simulink library "RGP_regression"  (R2020a)
settings: Solver=VariableStepAuto  StartTime=0.0  StopTime=10.0  RelTol=1e-3
values from neighbouring files (symbols this model uses):
  basisCovMat = basisCovMat + tril(basisCovMat,-1)'    [RGP_regression_ts.m]
  basisVector = rgp.xBasis    [RGP_regression_ts.m]
  hyperParameters = [rgp.spatialCovAmp(:); rgp.spatialLengthScale(:)]    [RGP_regression_ts.m]
  meanFcnProperties = rgp.meanFnProps    [RGP_regression_ts.m]
  meanFcnVector = meanFunction(basisVector,0)    [RGP_regression_ts.m]
  noiseVariance = rgp.noiseVariance    [RGP_regression_ts.m]
libraries: dspsigops x2, dspmtrx3 x1
settings Model: Creator=Ayaz  LastModifiedBy=Ayaz

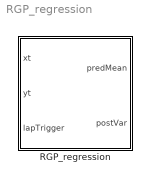
== system RGP_regression ==
  RGP_regression : Subsystem  mask{xBasis=basisVector, meanFcnProp=meanFcnProperties, meanFcnVec=meanFcnVector, hyperParams=hyperParameters, basisCovMat=basisCovMat, noiseVar=noiseVariance}
      mask prompts: xBasis "Basis vector"; meanFcnProp "Mean function properties"; meanFcnVec "Mean function vector"; hyperParams "Covariance hyperparameters"; basisCovMat "Basis vectors covariance matrix"; noiseVar "Noise variance"

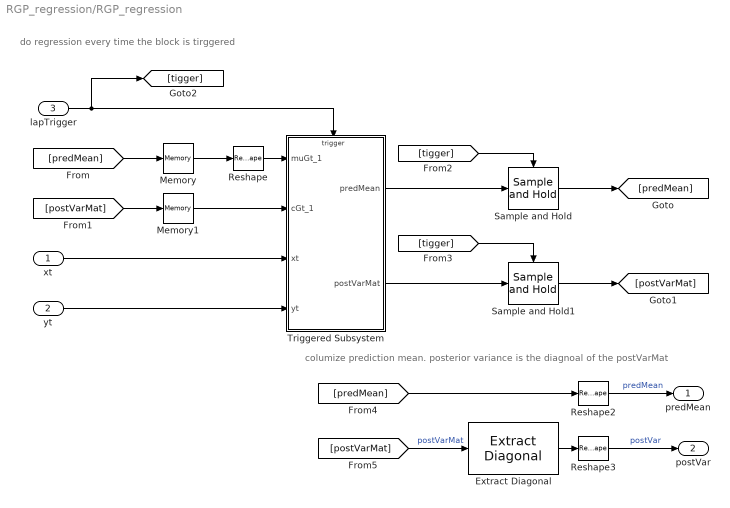
== system RGP_regression/RGP_regression ==
  note: columize prediction mean. posterior variance is the diagnoal of the postVarMat
  note: do regression every time the block is tirggered
  xt : Inport
  yt : Inport  Port=2
  lapTrigger : Inport  Port=3
  Extract Diagonal : dspmtrx3/Extract Diagonal
      settings: SourceProductBaseCode=DS
  Memory : Memory  InitialCondition=meanFcnVec
  Memory1 : Memory  InitialCondition=basisCovMat
  Reshape : Reshape  OutputDimensionality=Row vector (2-D)
  Reshape2 : Reshape  OutputDimensionality=Column vector (2-D)
  Reshape3 : Reshape  OutputDimensionality=Column vector (2-D)
  Sample and Hold : dspsigops/Sample and Hold  trig=Rising edge  initCond=meanFcnVec  latchinput=off
  Sample and Hold1 : dspsigops/Sample and Hold  trig=Rising edge  initCond=basisCovMat  latchinput=off
  Triggered Subsystem : Subsystem  TreatAsAtomicUnit=on
  predMean : Outport
  postVar : Outport  Port=2
  wires:
  [predMean] -> Memory/1
  [postVarMat] -> Memory1/1
  xt/1 -> Triggered Subsystem/3(xt)
  yt/1 -> Triggered Subsystem/4(yt)
  lapTrigger/1 -> [tigger], Triggered Subsystem/Trigger
  Memory/1 -> Reshape/1
  Memory1/1 -> Triggered Subsystem/2(cGt_1)
  Sample and Hold1/1 -> [postVarMat]
  Reshape/1 -> Triggered Subsystem/1(muGt_1)
  Sample and Hold/1 -> [predMean]
  Triggered Subsystem/2(postVarMat) -> Sample and Hold1/1
  Triggered Subsystem/1(predMean) -> Sample and Hold/1
  [tigger] -> Sample and Hold/Trigger
  [tigger] -> Sample and Hold1/Trigger
  [postVarMat] -> Extract Diagonal/1  "postVarMat"
  Extract Diagonal/1 -> Reshape3/1
  Reshape3/1 -> postVar/1  "postVar"
  [predMean] -> Reshape2/1
  Reshape2/1 -> predMean/1  "predMean"

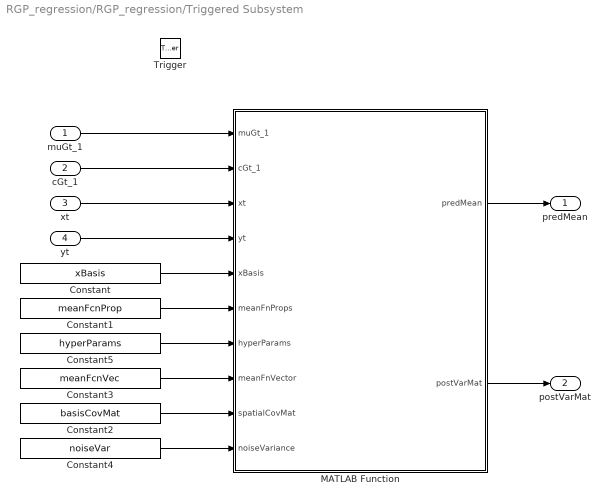
== system RGP_regression/RGP_regression/Triggered Subsystem ==
  muGt_1 : Inport
  cGt_1 : Inport  Port=2
  xt : Inport  Port=3
  yt : Inport  Port=4
  Trigger : TriggerPort  VariantControl=Variant
  Constant : Constant  Value=xBasis  VectorParams1D=off
  Constant1 : Constant  Value=meanFcnProp  VectorParams1D=off
  Constant2 : Constant  Value=basisCovMat  VectorParams1D=off
  Constant3 : Constant  Value=meanFcnVec  VectorParams1D=off
  Constant4 : Constant  Value=noiseVar  VectorParams1D=off
  Constant5 : Constant  Value=hyperParams  VectorParams1D=off
  MATLAB Function : MATLAB Function  TreatAsAtomicUnit=on
  predMean : Outport
  postVarMat : Outport  Port=2
  wires:
  Constant/1 -> MATLAB Function/5(xBasis)
  Constant1/1 -> MATLAB Function/6(meanFnProps)
  Constant3/1 -> MATLAB Function/8(meanFnVector)
  Constant2/1 -> MATLAB Function/9(spatialCovMat)
  Constant4/1 -> MATLAB Function/10(noiseVariance)
  muGt_1/1 -> MATLAB Function/1(muGt_1)
  cGt_1/1 -> MATLAB Function/2(cGt_1)
  xt/1 -> MATLAB Function/3(xt)
  yt/1 -> MATLAB Function/4(yt)
  MATLAB Function/1(predMean) -> predMean/1
  MATLAB Function/2(postVarMat) -> postVarMat/1
  Constant5/1 -> MATLAB Function/7(hyperParams)

== matlab function RGP_regression/Triggered Subsystem/MATLAB Function ==
  data: muGt_1 input; predMean output; cGt_1 input; xt input; yt input; xBasis input; meanFnProps input; hyperParams input; meanFnVector input; spatialCovMat input; noiseVariance input; postVarMat output
function [predMean,postVarMat] = calcPredMeanAndPostVar(...
    muGt_1,cGt_1,xt,yt,...%signals
    xBasis,meanFnProps,hyperParams,... % parameters
    meanFnVector,spatialCovMat,noiseVariance)

[predMean,postVarMat] = ...
    calcPredMeanAndPostVar(muGt_1,cGt_1,xt,yt,...%signals
    xBasis,meanFnProps,hyperParams,...
    meanFnVector,spatialCovMat,noiseVariance); % parameters

end
